simulink model "Continuous_Time_Design"  (R2024b)
settings: Solver=FixedStepAuto  StartTime=0.0  StopTime=10  FixedStep=0.01  RelTol=1e-3
libraries: slpidlib x3, simulink x1
(part 2 of 4)

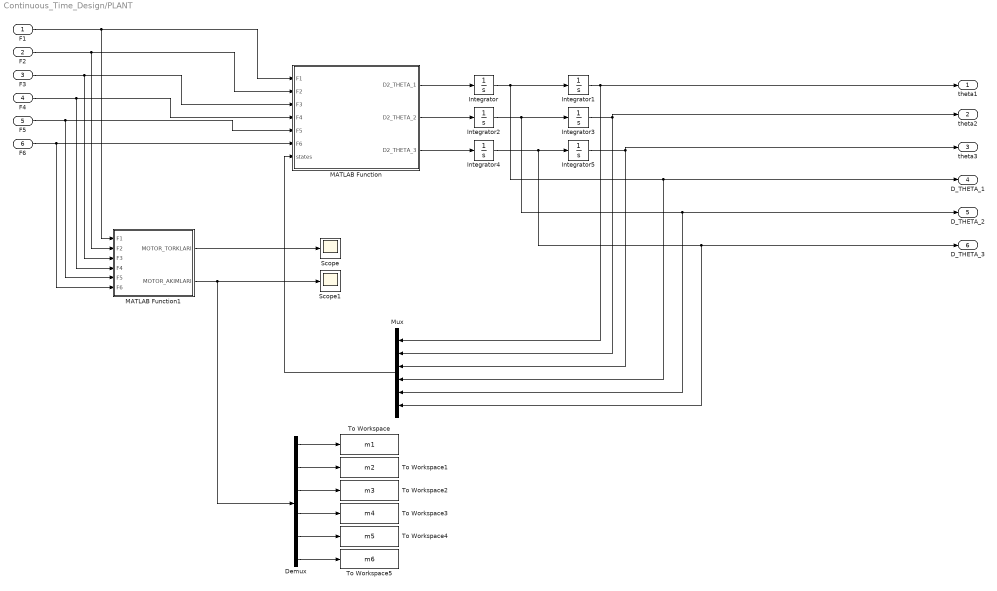
== system Continuous_Time_Design/PLANT ==
  F1 : Inport
  F2 : Inport  Port=2
  F3 : Inport  Port=3
  F4 : Inport  Port=4
  F5 : Inport  Port=5
  F6 : Inport  Port=6
  Demux : Demux  Outputs=6
  Integrator{,1..5} (6 alike) : Integrator
  MATLAB Function : MATLAB Function  TreatAsAtomicUnit=on
  MATLAB Function1 : MATLAB Function  TreatAsAtomicUnit=on
  Mux : Mux  Inputs=6
  Scope : Scope
  Scope1 : Scope
  To Workspace : ToWorkspace  VariableName=m1  SaveFormat=Timeseries  SampleTime=-1
  To Workspace1 : ToWorkspace  VariableName=m2  SaveFormat=Timeseries  SampleTime=-1
  To Workspace2 : ToWorkspace  VariableName=m3  SaveFormat=Timeseries  SampleTime=-1
  To Workspace3 : ToWorkspace  VariableName=m4  SaveFormat=Timeseries  SampleTime=-1
  To Workspace4 : ToWorkspace  VariableName=m5  SaveFormat=Timeseries  SampleTime=-1
  To Workspace5 : ToWorkspace  VariableName=m6  SaveFormat=Timeseries  SampleTime=-1
  theta1 : Outport
  theta2 : Outport  Port=2
  theta3 : Outport  Port=3
  D_THETA_1 : Outport  Port=4
  D_THETA_2 : Outport  Port=5
  D_THETA_3 : Outport  Port=6
  wires:
  MATLAB Function/1(D2_THETA_1) -> Integrator/1
  MATLAB Function/2(D2_THETA_2) -> Integrator2/1
  MATLAB Function/3(D2_THETA_3) -> Integrator4/1
  Integrator/1 -> Integrator1/1, Mux/4, D_THETA_1/1
  Integrator2/1 -> Mux/5, D_THETA_2/1, Integrator3/1
  Integrator4/1 -> Integrator5/1, Mux/6, D_THETA_3/1
  Integrator3/1 -> theta2/1, Mux/2
  Integrator5/1 -> theta3/1, Mux/3
  F1/1 -> MATLAB Function1/1(F1), MATLAB Function/1(F1)
  F2/1 -> MATLAB Function/2(F2), MATLAB Function1/2(F2)
  F3/1 -> MATLAB Function/3(F3), MATLAB Function1/3(F3)
  F4/1 -> MATLAB Function/4(F4), MATLAB Function1/4(F4)
  Mux/1 -> MATLAB Function/7(states)
  Integrator1/1 -> theta1/1, Mux/1
  F5/1 -> MATLAB Function/5(F5), MATLAB Function1/5(F5)
  F6/1 -> MATLAB Function/6(F6), MATLAB Function1/6(F6)
  MATLAB Function1/1(MOTOR_TORKLARI) -> Scope/1
  Demux/1 -> To Workspace/1
  MATLAB Function1/2(MOTOR_AKIMLARI) -> Demux/1, Scope1/1
  Demux/2 -> To Workspace1/1
  Demux/3 -> To Workspace2/1
  Demux/4 -> To Workspace3/1
  Demux/5 -> To Workspace4/1
  Demux/6 -> To Workspace5/1

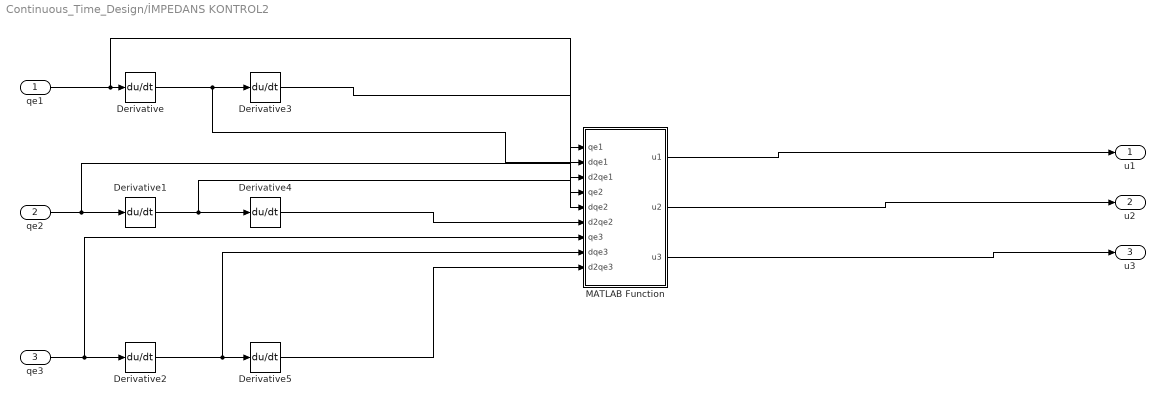
== system Continuous_Time_Design/İMPEDANS KONTROL2 ==
  qe1 : Inport
  qe2 : Inport  Port=2
  qe3 : Inport  Port=3
  Derivative{,1..5} (6 alike) : Derivative
  MATLAB Function : MATLAB Function  TreatAsAtomicUnit=on
  u1 : Outport
  u2 : Outport  Port=2
  u3 : Outport  Port=3
  wires:
  qe1/1 -> MATLAB Function/1(qe1), Derivative/1
  qe2/1 -> MATLAB Function/4(qe2), Derivative1/1
  qe3/1 -> MATLAB Function/7(qe3), Derivative2/1
  Derivative/1 -> MATLAB Function/2(dqe1), Derivative3/1
  Derivative1/1 -> MATLAB Function/5(dqe2), Derivative4/1
  Derivative2/1 -> MATLAB Function/8(dqe3), Derivative5/1
  Derivative3/1 -> MATLAB Function/3(d2qe1)
  Derivative4/1 -> MATLAB Function/6(d2qe2)
  Derivative5/1 -> MATLAB Function/9(d2qe3)
  MATLAB Function/1(u1) -> u1/1
  MATLAB Function/2(u2) -> u2/1
  MATLAB Function/3(u3) -> u3/1

== matlab function Continuous_Time_Design/PLANT/MATLAB Function1 ==
  data: F1 input; MOTOR_TORKLARI output; F2 input; F3 input; F4 input; F5 input; F6 input; MOTOR_AKIMLARI output
function [MOTOR_TORKLARI, MOTOR_AKIMLARI] = fcn(F1, F2, F3, F4, F5, F6)

m1t = F1*0.0125;
m2t = F2*0.0125;
m3t = F3*0.0125;

m4t = F4*0.0125;
m5t = F5*0.0125;
m6t = F6*0.0125;

MOTOR_TORKLARI = [m1t; m2t; m3t; m4t; m5t; m6t];
MOTOR_AKIMLARI = [m1t/0.87; m2t/0.87; m3t/0.87; m4t/0.87; m5t/0.87; m6t/0.87];
end
